simulink model "ncp_spectrum_sl"  (R2018b)
settings: Solver=VariableStepAuto  StartTime=0.0  StopTime=10  RelTol=1e-3  EnableMultiTasking=on
PreLoadFcn:
  | addpath('../')
settings Model: Creator=user  LastModifiedBy=abartolome
settings OptimizationCC: LifeSpan=inf
settings DebuggingCC: SFUnexpectedBacktrackingDiag=warning  SFNoUnconditionalDefaultTransitionDiag=warning
settings SFSimCC: SimUseLocalCustomCode=off
settings RTWCC: RTWUseLocalCustomCode=off
settings CodeAppCC: StateflowObjectComments=on
settings GRTTargetCC: TargetLangStandard=C89/C90 (ANSI)  GeneratePreprocessorConditionals=Disable all
settings ConfigComp: CovMetricSettings=dw  CovHtmlReporting=on  CovSaveCumulativeToWorkspaceVar=on  CovSaveSingleToWorkspaceVar=on  CovExternalEMLEnable=off

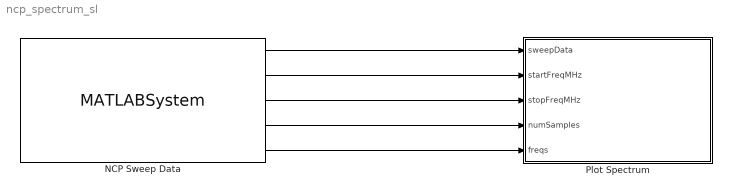
== system ncp_spectrum_sl ==
  "NCP Sweep Data " : MATLABSystem  StopFcn=|  System=ncp_sweep_data  startFreqMHzReq=900  stopFreqMHzReq=920  bandwidthHz=200000  node_ip=192.0.2.0  node_port=9999  SimulateUsing=Interpreted execution
      | if libisloaded('matlab_ncp_lib')
      |   calllib('matlab_ncp_lib', 'EndSweep');
      |   unloadlibrary('matlab_ncp_lib');
      | end
      mask Type: ncp_sweep_data
      mask Display:
      | disp('ncp_sweep_data');
      | port_label('output',1,'sweepData');
      | port_label('output',2,'startFreqMHz');
      | port_label('output',3,'stopFreqMHz');
      | port_label('output',4,'numSamples');
      | port_label('output',5,'freqs');
  Plot Spectrum : MATLAB Function  TreatAsAtomicUnit=on
  wires:
  "NCP Sweep Data "/1 -> Plot Spectrum/1(sweepData)
  "NCP Sweep Data "/2 -> Plot Spectrum/2(startFreqMHz)
  "NCP Sweep Data "/4 -> Plot Spectrum/4(numSamples)
  "NCP Sweep Data "/3 -> Plot Spectrum/3(stopFreqMHz)
  "NCP Sweep Data "/5 -> Plot Spectrum/5(freqs)

== matlab function ncp_spectrum_sl/Plot Spectrum ==
  data: sweepData input; startFreqMHz input; stopFreqMHz input; numSamples input; freqs input
function plot_spec(sweepData,startFreqMHz,stopFreqMHz,numSamples,freqs)

% Plot spectrum
plot(freqs(1:numSamples),sweepData(1:numSamples),'y');
set(gca,'Color','k')
%title(['Spectrum ' num2str(startFreqMHzReq) '-' num2str(stopFreqMHzReq) ' MHz '...
%    '(' num2str(bandwidthHz) ' Hz resolution BW)']);
xlim([startFreqMHz stopFreqMHz]);
xlabel('Frequency (MHz)');
ylabel('Power (dBm)');
